simulink model "lab5_ASP_BolonkinaA"  (R2018b)
settings: Solver=VariableStepAuto  StartTime=0.0  StopTime=10.0  RelTol=1e-3
libraries: dspsrcs4 x2, dspsnks4 x1, dspvision x1
settings Model: Creator=Student  LastModifiedBy=Student

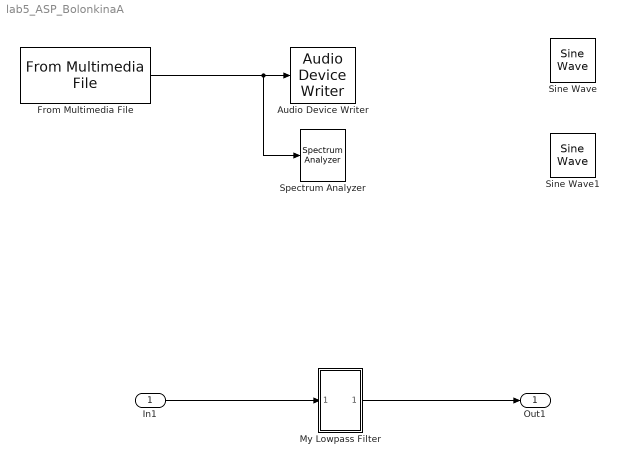
== system lab5_ASP_BolonkinaA ==
  In1 : Inport
  Audio Device Writer : dspsnks4/Audio Device Writer  Driver=DirectSound  Device=Default  InheritSampleRate=on  SampleRate=44100  BitDepth=16-bit integer  BufferSize=4096  NumBuffers=10  DefaultOutputChannelMapping=on  OutputChannelMapping=1:2  OutputNumUnderrunSamples=off  DriverIdx=1  DeviceWarnFlag=''
  From Multimedia File : dspvision/From Multimedia File  inputFilename=C:\Users\student\Documents\MATLAB\song.mp3  loop=on  numPlays=inf  outputStreams=Audio only  videoDataType=single  audioDataType=double  inheritSampleTime=on  userDefinedSampleTime=1/30  noAudioOutput=off  isIntensityVideo=off  fourcc=RGB  colorVideoFormat=Separate color signals  outputEOF=off  dataOrg=Column-major  audioFrameSize=1024  computeAudioFrameSize=off  outSamplingMode=Sample based
      settings: SourceProductBaseCode=VP
  My Lowpass Filter : Subsystem
  Sine Wave : dspsrcs4/Sine Wave  Amplitude=1  Frequency=17000  Phase=0  SampleMode=Discrete  OutComplex=Real  CompMethod=Trigonometric fcn  TableSize=Speed  SampleTime=1/44100  SamplesPerFrame=1024  ResetState=Restart at time zero  OutputFrames=off  dataType=double  wordLen=16  udDataType=sfix(16)  fracBitsMode=Best precision  numFracBits=15  OutDataTypeStr=double  LastOutDataTypeStr=double
  Sine Wave1 : dspsrcs4/Sine Wave  Amplitude=1  Frequency=17000  Phase=0  SampleMode=Discrete  OutComplex=Real  CompMethod=Trigonometric fcn  TableSize=Speed  SampleTime=1/44100  SamplesPerFrame=1024  ResetState=Restart at time zero  OutputFrames=off  dataType=double  wordLen=16  udDataType=sfix(16)  fracBitsMode=Best precision  numFracBits=15  OutDataTypeStr=double  LastOutDataTypeStr=double
  Spectrum Analyzer : SpectrumAnalyzer
  Out1 : Outport
  wires:
  From Multimedia File/1 -> Spectrum Analyzer/1, Audio Device Writer/1
  In1/1 -> My Lowpass Filter/1(In1)
  My Lowpass Filter/1(Out1) -> Out1/1

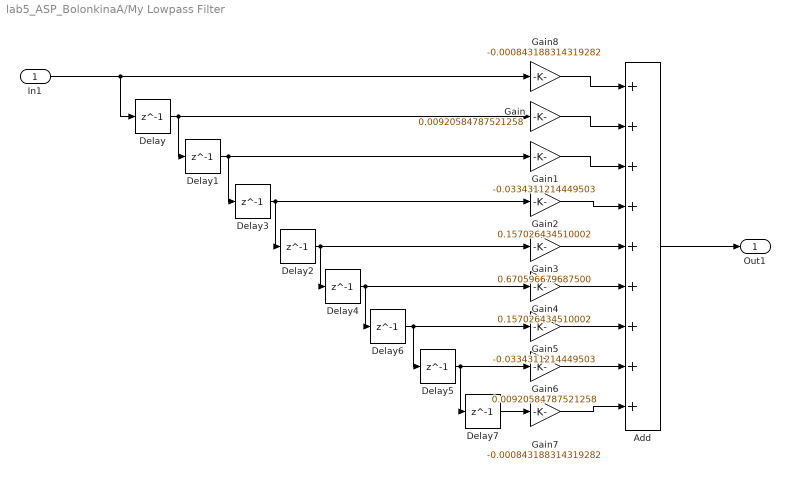
== system lab5_ASP_BolonkinaA/My Lowpass Filter ==
  In1 : Inport
  Add : Sum  Inputs=+++++++++
  Delay{,1..7} (8 alike) : Delay  DelayLength=1  InitialCondition=0
  Gain : Gain  Gain=0.00920584787521258
  Gain1 : Gain  Gain=-0.0334311214449503
  Gain2 : Gain  Gain=0.157026434510002
  Gain3 : Gain  Gain=0.670596679687500
  Gain4 : Gain  Gain=0.157026434510002
  Gain5 : Gain  Gain=-0.0334311214449503
  Gain6 : Gain  Gain=0.00920584787521258
  Gain7 : Gain  Gain=-0.000843188314319282
  Gain8 : Gain  Gain=-0.000843188314319282
  Out1 : Outport
  wires:
  Gain4/1 -> Add/6
  In1/1 -> Delay/1, Gain8/1
  Delay3/1 -> Gain2/1, Delay2/1
  Delay6/1 -> Gain5/1, Delay5/1
  Gain/1 -> Add/2
  Delay1/1 -> Gain1/1, Delay3/1
  Gain6/1 -> Add/8
  Delay4/1 -> Gain4/1, Delay6/1
  Gain8/1 -> Add/1
  Gain5/1 -> Add/7
  Delay/1 -> Gain/1, Delay1/1
  Delay2/1 -> Gain3/1, Delay4/1
  Delay5/1 -> Gain6/1, Delay7/1
  Gain1/1 -> Add/3
  Gain7/1 -> Add/9
  Gain2/1 -> Add/4
  Delay7/1 -> Gain7/1
  Gain3/1 -> Add/5
  Add/1 -> Out1/1
